simulink library "Actuator_Lib"  (Simulink 8.4)
settings: Solver=ode45  StartTime=0.0  StopTime=10.0  RelTol=1e-3
values from neighbouring files (symbols this model uses):
  AC = miniMUTT_rigid_config    [UAV_config.m]    (also in UAV_modelconfig.mat = )
  TrimCondition =     [UAV_trimcondition.mat]
undefined symbols (not defined in the file or in its folder): SampleTime
libraries: Actuator_Lib x31, simulink x7
settings Model: RequirementInfo="{}  %GIDa_26eb398f_e494_4241_9189_ccb3fdb74222"  Creator=austinmurch  LastModifiedBy=pseiler

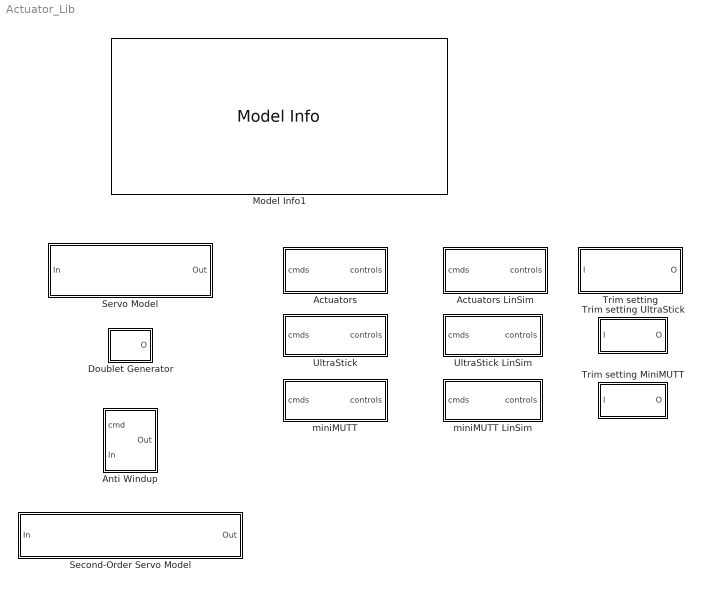
== system Actuator_Lib ==
  Actuators : Subsystem  BlockChoice=UltraStick  mask{aircraft=AC.aircraft}
      mask help: Set actuator models, either 'UltraStick120', 'UltraStick25e', or 'miniMUTT'
      mask init:
      | pathname = gcb;
      | 
      | switch lower(aircraft)
      |     case 'ultrastick120'
      |         set_param(pathname,'BlockChoice','UltraStick');
      |     case 'ultrastick25e'
      |         set_param(pathname,'BlockChoice','UltraStick');
      |     case 'minimutt'
      |         set_param(pathname,'BlockChoice','miniMUTT');
      |     case 'rigid_minimutt'
      |         set_param(pathname,'BlockChoice','miniMUTT');
      | end
      settings: TemplateBlock=self  MemberBlocks=UltraStick,miniMUTT
  Actuators LinSim : Subsystem  BlockChoice=miniMUTT LinSim  mask{aircraft=AC.aircraft}
      mask help: Set actuator models, either 'UltraStick120', 'UltraStick25e', or 'miniMUTT'
      mask init:
      | pathname = gcb;
      | 
      | switch lower(aircraft)
      |     case 'ultrastick120'
      |         set_param(pathname,'BlockChoice','UltraStick LinSim');
      |     case 'ultrastick25e'
      |         set_param(pathname,'BlockChoice','UltraStick LinSim');
      |     case 'minimutt'
      |         set_param(pathname,'BlockChoice','miniMUTT LinSim');
      |     case 'rigid_minimutt'
      |         set_param(pathname,'BlockChoice','miniMUTT LinSim');
      | end
      settings: TemplateBlock=self  MemberBlocks=UltraStick LinSim,miniMUTT LinSim
  Anti Windup : Subsystem  mask(Integrator Anti-Windup){MAX_DEF=0, MIN_DEF=0, gain_sign=off}
      mask prompts: MAX_DEF "Maximum surface deflection limit"; MIN_DEF "Minimum surface deflection limit"; gain_sign "Positive gains in control law"
      mask help:
      | This block uses boolean logic to eliminate integrator windup.
      | It compares the sign of the error between reference and output,
      | and the sign and position of the surface being controlled.
      mask Help:
      | See the "READ ME" block under the mask for a more thorough explanation of
      | how this block works.
  Doublet Generator : Subsystem  mask(DoubletGenerator){timeon=[3 10 17], pulsewidth=[2 2 2], amplitude=[0 0 0]}
      mask prompts: timeon "Time Start"; pulsewidth "Pulse Duration"
      mask help:
      | Doublet Generator.
      | Ouputs doublet of specificed amplitude and duration.
      |
      | If start/duration/amplitude parameters are vectors, then output is multichannel.
      mask Display: plot([.1 .3 .3001 .4 .4001 .5  .5001 .7],[0 0 1 1 -1 -1 0 0])
  Model Info1 : simulink/Model-Wide Utilities/Model Info  BlockCM=None  Frame=on  DisplayStringWithTags=|  HorizontalTextAlignment=Left  LeftAlignmentValue=0.02  SourceBlockDiagram=Actuator_Lib  TagMaxNumber=20
      | MODEL INFORMATION
      | Actuator Model Library
      | 
      | University of Minnesota
      | Aerospace Engineering and Mechanics
      | Copyright 2011 Regents of the University of Minnesota. All rights reserved.
      | 
      | == SVN Info ==
      | Last modified by %<LastModifiedBy> on %<LastModificationDate>
  Second-Order Servo Model : Subsystem  mask(Rate and Position Limited Servo){wn=10, zeta=1, RL=999, POS_hi=inf, POS_lo=-inf}
      mask prompts: wn "Natural Frequency, rad/sec"; zeta "Damping Ratio, unitless"; RL "Rate Limit:"; POS_hi "Position Limit High:"; POS_lo "Position Limit Low:"
      mask help: First order transfer function: w/(s+w), with rate and position limits.
      mask Help:
      | This block models a first order servo with the initial condition
      | on the integrator set to the steady state value for constant input.
      | The servo is rate and position limited and those values are set
      | in the block parameters.
      mask Display:
      | text(.48,.55,sprintf('wn=%3.1f rad/sec\n zeta= %3.1f',wn,zeta),'horizontalAlignment','center');
      | 
      | text(0.18,0.45,sprintf('|d/dt|\n<%0.1f',RL),'horizontalAlignment','center');
      | 
      | text(0.88,0.85,num2str(POS_hi),'horizontalAlignment', 'center');
      | text(0.88,0.2,num2str(POS_lo),'horizontalAlignment', 'center');
      | text(0.73,0.5,'P\nL');
      | 
      | 
      | plot([0.83 0.87 0.93 0.97],[0.4 0.4 0.6 0.6]);
      | plot([0.81 0.99],[0.5 0.5]);
      | plot([0.9 0.9],[0.3 0.7]);
      | plot([0.81 0.99 0.99 0.81 0.81],[0.3 0.3 0.7 0.7 0.3]);
  Servo Model : Subsystem  mask(Rate and Position Limited Servo){freq=10, RL=999.0, POS_hi=20.0, POS_lo=-30.0}
      mask prompts: freq "Bandwidth, Hz"; RL "Rate Limit:"; POS_hi "Position Limit High:"; POS_lo "Position Limit Low:"
      mask help: First order transfer function: w/(s+w), with rate and position limits.
      mask Help:
      | This block models a first order servo with the initial condition
      | on the integrator set to the steady state value for constant input.
      | The servo is rate and position limited and those values are set
      | in the block parameters.
      mask Display:
      | text(.48,.55,sprintf('%3.1f Hz\nBW',freq),'horizontalAlignment','center');
      | 
      | text(0.18,0.45,sprintf('|d/dt|\n<%0.1f',RL),'horizontalAlignment','center');
      | 
      | text(0.88,0.85,num2str(POS_hi),'horizontalAlignment', 'center');
      | text(0.88,0.2,num2str(POS_lo),'horizontalAlignment', 'center');
      | text(0.73,0.5,'P\nL');
      | 
      | 
      | plot([0.83 0.87 0.93 0.97],[0.4 0.4 0.6 0.6]);
      | plot([0.81 0.99],[0.5 0.5]);
      | plot([0.9 0.9],[0.3 0.7]);
      | plot([0.81 0.99 0.99 0.81 0.81],[0.3 0.3 0.7 0.7 0.3]);
  Trim setting : Subsystem  RequirementInfo="{}  %GIDa_fb3b993e_8e22_4fb1_9c4b_299134347a17"  BlockChoice=Trim setting UltraStick  mask{aircraft=AC.aircraft}
      mask prompts: aircraft "Aircraft model"
      mask init:
      | pathname = gcb;
      | 
      | switch lower(aircraft)
      |     case 'ultrastick120'
      |         set_param(pathname,'BlockChoice','Trim setting UltraStick');
      |     case 'ultrastick25e'
      |         set_param(pathname,'BlockChoice','Trim setting UltraStick');
      |     case 'minimutt'
      |         set_param(pathname,'BlockChoice','Trim setting MiniMUTT');
      |     case 'rigid_minimutt'
      |         set_param(pathname,'BlockChoice','Trim setting MiniMUTT');
      | end
      settings: TemplateBlock=self  MemberBlocks=Trim setting MiniMUTT,Trim setting UltraStick
  Trim setting MiniMUTT : Subsystem
  Trim setting UltraStick : Subsystem
  UltraStick : Subsystem
  UltraStick LinSim : Subsystem
  miniMUTT : Subsystem
  miniMUTT LinSim : Subsystem

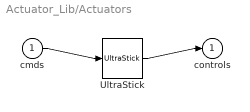
== system Actuator_Lib/Actuators ==
  cmds : Inport
  UltraStick : Actuator_Lib/UltraStick
  controls : Outport
  wires:
  cmds/1 -> UltraStick/1
  UltraStick/1 -> controls/1

== system Actuator_Lib/Actuators LinSim ==
  cmds : Inport
  miniMUTT LinSim : Actuator_Lib/miniMUTT LinSim
  controls : Outport
  wires:
  cmds/1 -> miniMUTT LinSim/1
  miniMUTT LinSim/1 -> controls/1

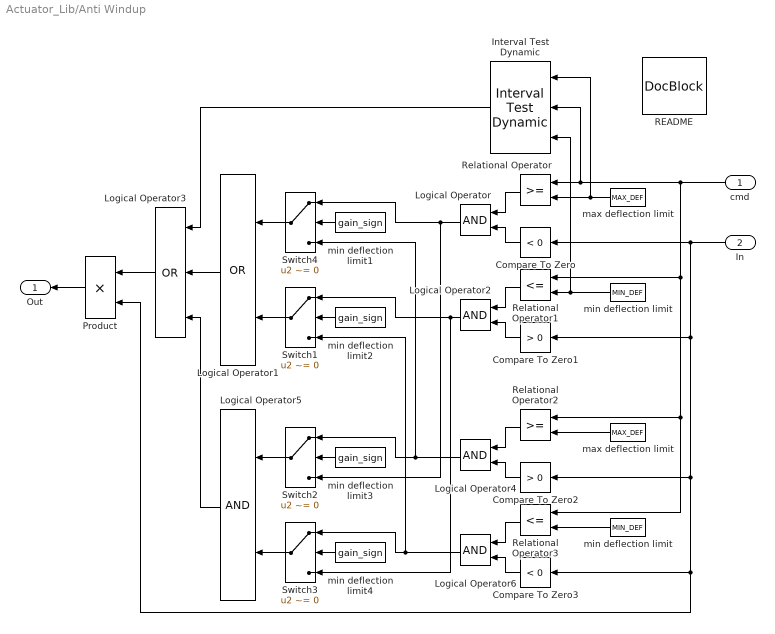
== system Actuator_Lib/Anti Windup ==
  cmd : Inport
  In : Inport  Port=2
  Compare To Zero : simulink/Logic and Bit Operations/Compare To Zero  relop=<  OutDataTypeStr=uint8
  Compare To Zero1 : simulink/Logic and Bit Operations/Compare To Zero  relop=>  OutDataTypeStr=uint8
  Compare To Zero2 : simulink/Logic and Bit Operations/Compare To Zero  relop=>  OutDataTypeStr=uint8
  Compare To Zero3 : simulink/Logic and Bit Operations/Compare To Zero  relop=<  OutDataTypeStr=uint8
  Interval Test Dynamic : simulink/Logic and Bit Operations/Interval Test Dynamic  IntervalClosedRight=on  IntervalClosedLeft=on  OutDataTypeStr=boolean
  Logical Operator{,2,4..6} (5 alike) : Logic  AllPortsSameDT=off  OutDataTypeStr=boolean  SampleTime=SampleTime
  Logical Operator1 : Logic  Operator=OR  AllPortsSameDT=off  OutDataTypeStr=boolean  SampleTime=SampleTime
  Logical Operator3 : Logic  Operator=OR  Inputs=3  AllPortsSameDT=off  OutDataTypeStr=boolean  SampleTime=SampleTime
  Product : Product  RndMeth=Zero
  README : simulink/Model-Wide Utilities/DocBlock  DocumentType=Text
  Relational Operator : RelationalOperator  OutDataTypeStr=boolean
  Relational Operator1 : RelationalOperator  Operator=<=  OutDataTypeStr=boolean
  Relational Operator2 : RelationalOperator  OutDataTypeStr=boolean
  Relational Operator3 : RelationalOperator  Operator=<=  OutDataTypeStr=boolean
  Switch{1..4} (4 alike) : Switch  Criteria=u2 ~= 0  SampleTime=SampleTime
  max deflection limit : Constant  Value=MAX_DEF  SampleTime=SampleTime
  "max deflection limit " : Constant  Value=MAX_DEF  SampleTime=SampleTime
  min deflection limit : Constant  Value=MIN_DEF  SampleTime=SampleTime
  "min deflection limit " : Constant  Value=MIN_DEF  SampleTime=SampleTime
  min deflection limit{1..4} (4 alike) : Constant  Value=gain_sign  SampleTime=SampleTime
  Out : Outport
  wires:
  Logical Operator5/1 -> Logical Operator3/3
  "max deflection limit "/1 -> Relational Operator2/2
  "min deflection limit "/1 -> Relational Operator3/2
  Relational Operator3/1 -> Logical Operator6/1
  Compare To Zero3/1 -> Logical Operator6/2
  Relational Operator2/1 -> Logical Operator4/1
  Compare To Zero2/1 -> Logical Operator4/2
  Interval Test Dynamic/1 -> Logical Operator3/1
  Logical Operator1/1 -> Logical Operator3/2
  Logical Operator3/1 -> Product/1
  Product/1 -> Out/1
  min deflection limit/1 -> Interval Test Dynamic/3, Relational Operator1/2
  Relational Operator1/1 -> Logical Operator2/1
  Compare To Zero1/1 -> Logical Operator2/2
  In/1 -> Product/2, Compare To Zero3/1, Compare To Zero2/1, Compare To Zero1/1, Compare To Zero/1
  Relational Operator/1 -> Logical Operator/1
  Compare To Zero/1 -> Logical Operator/2
  cmd/1 -> Relational Operator3/1, Relational Operator2/1, Relational Operator1/1, Interval Test Dynamic/2, Relational Operator/1
  max deflection limit/1 -> Interval Test Dynamic/1, Relational Operator/2
  min deflection limit2/1 -> Switch1/2
  min deflection limit3/1 -> Switch2/2
  min deflection limit4/1 -> Switch3/2
  Switch2/1 -> Logical Operator5/1
  Switch3/1 -> Logical Operator5/2
  Switch1/1 -> Logical Operator1/2
  Switch4/1 -> Logical Operator1/1
  min deflection limit1/1 -> Switch4/2
  Logical Operator/1 -> Switch4/1, Switch2/3
  Logical Operator2/1 -> Switch1/1, Switch3/3
  Logical Operator4/1 -> Switch2/1, Switch4/3
  Logical Operator6/1 -> Switch3/1, Switch1/3

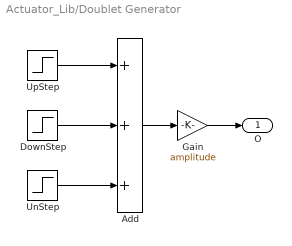
== system Actuator_Lib/Doublet Generator ==
  Add : Sum  Inputs=+++
  DownStep : Step  Time=timeon+pulsewidth  After=-2  SampleTime=0
  Gain : Gain  Gain=amplitude
  UnStep : Step  Time=timeon+2*pulsewidth  SampleTime=0
  UpStep : Step  Time=timeon  SampleTime=0
  O : Outport
  wires:
  Gain/1 -> O/1
  Add/1 -> Gain/1
  UnStep/1 -> Add/3
  DownStep/1 -> Add/2
  UpStep/1 -> Add/1

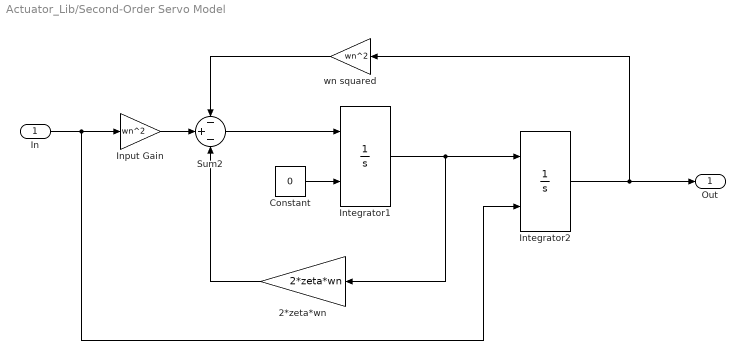
== system Actuator_Lib/Second-Order Servo Model ==
  In : Inport
  2*zeta*wn : Gain  Gain=2*zeta*wn
  Constant : Constant  Value=0
  Input Gain : Gain  Gain=wn^2
  Integrator1 : Integrator  InitialConditionSource=external  LimitOutput=on  UpperSaturationLimit=RL  LowerSaturationLimit=-RL  IgnoreLimit=on
  Integrator2 : Integrator  InitialConditionSource=external  LimitOutput=on  UpperSaturationLimit=POS_hi  LowerSaturationLimit=POS_lo  IgnoreLimit=on
  Sum2 : Sum  Inputs=-+-
  wn squared : Gain  Gain=wn^2
  Out : Outport  PortDimensions=1
  wires:
  In/1 -> Input Gain/1, Integrator2/2
  Input Gain/1 -> Sum2/2
  2*zeta*wn/1 -> Sum2/3
  Constant/1 -> Integrator1/2
  Sum2/1 -> Integrator1/1
  Integrator1/1 -> Integrator2/1, 2*zeta*wn/1
  wn squared/1 -> Sum2/1
  Integrator2/1 -> Out/1, wn squared/1

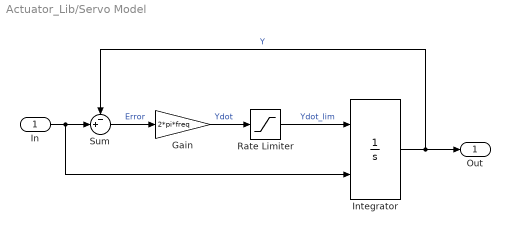
== system Actuator_Lib/Servo Model ==
  In : Inport
  Gain : Gain  Gain=2*pi*freq  SaturateOnIntegerOverflow=on  OutDataTypeStr=Inherit: Same as input  ParamDataTypeStr=Inherit: Same as input
  Integrator : Integrator  InitialConditionSource=external  LimitOutput=on  UpperSaturationLimit=POS_hi  LowerSaturationLimit=POS_lo  IgnoreLimit=on
  Rate Limiter : Saturate  UpperLimit=RL  LowerLimit=-RL
  Sum : Sum  Inputs=-+|  SaturateOnIntegerOverflow=on  InputSameDT=on  OutDataTypeStr=Inherit: Same as first input
  Out : Outport  PortDimensions=1
  wires:
  Gain/1 -> Rate Limiter/1  "Ydot"
  Sum/1 -> Gain/1  "Error"
  Integrator/1 -> Sum/1, Out/1  "Y"
  Rate Limiter/1 -> Integrator/1  "Ydot_lim"
  In/1 -> Integrator/2, Sum/2

== system Actuator_Lib/Trim setting ==
  I : Inport
  Trim setting UltraStick : Actuator_Lib/Trim setting UltraStick
  O : Outport
  wires:
  I/1 -> Trim setting UltraStick/1
  Trim setting UltraStick/1 -> O/1

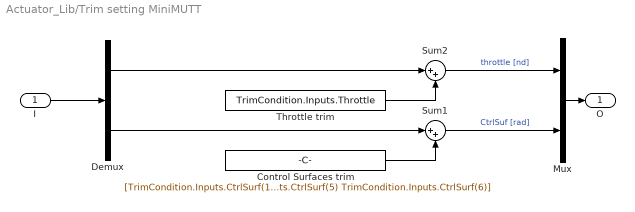
== system Actuator_Lib/Trim setting MiniMUTT ==
  I : Inport
  Control Surfaces trim : Constant  Value=[TrimCondition.Inputs.CtrlSurf(1) TrimCondition.Inputs.CtrlSurf(2) TrimCondition.Inputs.CtrlSurf(3) TrimCondition.Inputs.CtrlSurf(4) TrimCondition.Inputs.CtrlSurf(5) TrimCondition.Inputs.CtrlSurf(6)]
  Demux : Demux  Outputs=[1 ,-1]
  Mux : Mux  Inputs=2
  Sum1 : Sum  Inputs=|++
  Sum2 : Sum  Inputs=|++
  Throttle trim : Constant  Value=TrimCondition.Inputs.Throttle
  O : Outport
  wires:
  Sum1/1 -> Mux/2  "CtrlSuf [rad]"
  Demux/1 -> Sum2/1
  Sum2/1 -> Mux/1  "throttle [nd]"
  Throttle trim/1 -> Sum2/2
  Control Surfaces trim/1 -> Sum1/2
  I/1 -> Demux/1
  Demux/2 -> Sum1/1
  Mux/1 -> O/1

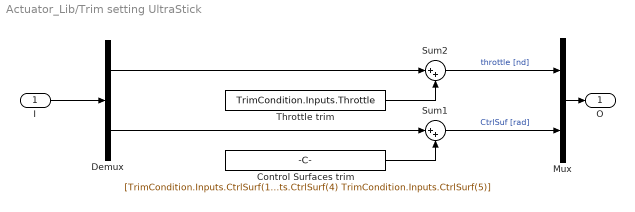
== system Actuator_Lib/Trim setting UltraStick ==
  I : Inport
  Control Surfaces trim : Constant  Value=[TrimCondition.Inputs.CtrlSurf(1) TrimCondition.Inputs.CtrlSurf(2) TrimCondition.Inputs.CtrlSurf(3)*-1 TrimCondition.Inputs.CtrlSurf(3) TrimCondition.Inputs.CtrlSurf(4) TrimCondition.Inputs.CtrlSurf(5)]
  Demux : Demux  Outputs=[1 ,-1]
  Mux : Mux  Inputs=2
  Sum1 : Sum  Inputs=|++
  Sum2 : Sum  Inputs=|++
  Throttle trim : Constant  Value=TrimCondition.Inputs.Throttle
  O : Outport
  wires:
  Sum1/1 -> Mux/2  "CtrlSuf [rad]"
  Demux/1 -> Sum2/1
  Sum2/1 -> Mux/1  "throttle [nd]"
  Throttle trim/1 -> Sum2/2
  Control Surfaces trim/1 -> Sum1/2
  I/1 -> Demux/1
  Demux/2 -> Sum1/1
  Mux/1 -> O/1

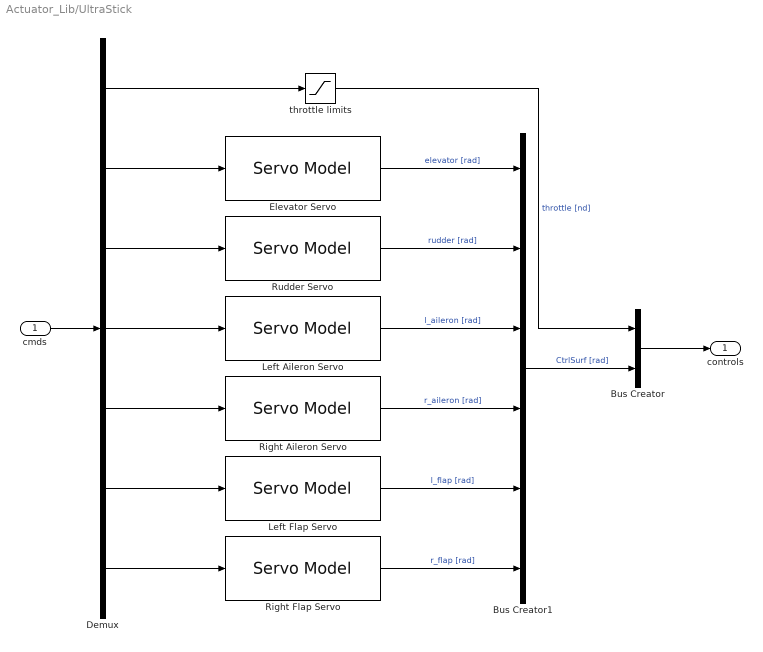
== system Actuator_Lib/UltraStick ==
  cmds : Inport
  Bus Creator : BusCreator  Inputs=2
  Bus Creator1 : BusCreator  Inputs=6
  Demux : Demux  Outputs=7
  Elevator Servo : Actuator_Lib/Servo Model  freq=AC.Actuator.elevator.BW  RL=AC.Actuator.elevator.RateLim  POS_hi=AC.Actuator.elevator.PosLim  POS_lo=AC.Actuator.elevator.NegLim
  Left Aileron Servo : Actuator_Lib/Servo Model  freq=AC.Actuator.l_aileron.BW  RL=AC.Actuator.l_aileron.RateLim  POS_hi=AC.Actuator.l_aileron.PosLim  POS_lo=AC.Actuator.l_aileron.NegLim
  Left Flap Servo : Actuator_Lib/Servo Model  freq=AC.Actuator.l_flap.BW  RL=AC.Actuator.l_flap.RateLim  POS_hi=AC.Actuator.l_flap.PosLim  POS_lo=AC.Actuator.l_flap.NegLim
  Right Aileron Servo : Actuator_Lib/Servo Model  freq=AC.Actuator.r_aileron.BW  RL=AC.Actuator.r_aileron.RateLim  POS_hi=AC.Actuator.r_aileron.PosLim  POS_lo=AC.Actuator.r_aileron.NegLim
  Right Flap Servo : Actuator_Lib/Servo Model  freq=AC.Actuator.l_flap.BW  RL=AC.Actuator.l_flap.RateLim  POS_hi=AC.Actuator.l_flap.PosLim  POS_lo=AC.Actuator.l_flap.NegLim
  Rudder Servo : Actuator_Lib/Servo Model  freq=AC.Actuator.rudder.BW  RL=AC.Actuator.rudder.RateLim  POS_hi=AC.Actuator.rudder.PosLim  POS_lo=AC.Actuator.rudder.NegLim
  throttle limits : Saturate  UpperLimit=AC.Actuator.throttle.PosLim  LowerLimit=AC.Actuator.throttle.NegLim
  controls : Outport
  wires:
  Demux/5 -> Right Aileron Servo/1
  Demux/7 -> Right Flap Servo/1
  Right Flap Servo/1 -> Bus Creator1/6  "r_flap [rad]"
  Right Aileron Servo/1 -> Bus Creator1/4  "r_aileron [rad]"
  Left Flap Servo/1 -> Bus Creator1/5  "l_flap [rad]"
  Demux/6 -> Left Flap Servo/1
  Left Aileron Servo/1 -> Bus Creator1/3  "l_aileron [rad]"
  Demux/4 -> Left Aileron Servo/1
  Rudder Servo/1 -> Bus Creator1/2  "rudder [rad]"
  Demux/3 -> Rudder Servo/1
  Elevator Servo/1 -> Bus Creator1/1  "elevator [rad]"
  Demux/2 -> Elevator Servo/1
  throttle limits/1 -> Bus Creator/1  "throttle [nd]"
  Demux/1 -> throttle limits/1
  cmds/1 -> Demux/1
  Bus Creator/1 -> controls/1
  Bus Creator1/1 -> Bus Creator/2  "CtrlSurf [rad]"

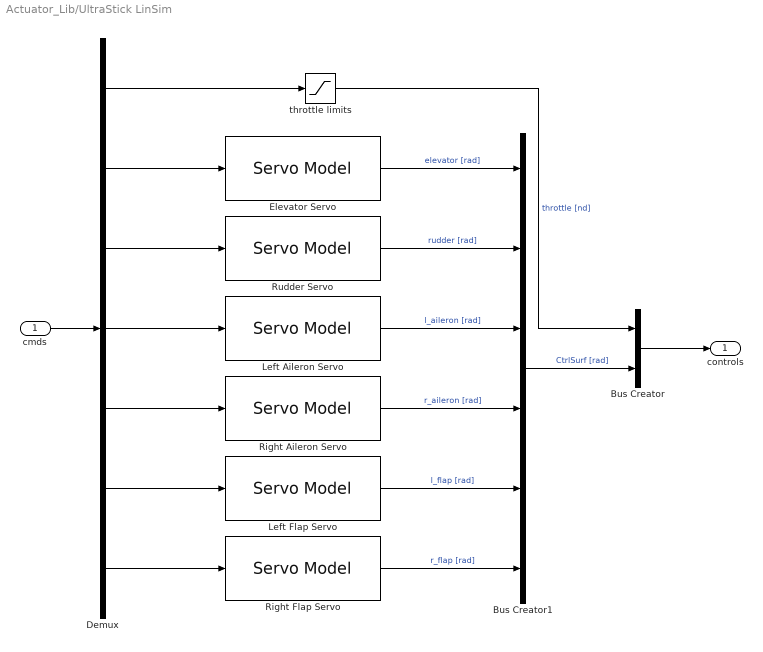
== system Actuator_Lib/UltraStick LinSim ==
  cmds : Inport
  Bus Creator : BusCreator  Inputs=2
  Bus Creator1 : BusCreator  Inputs=6
  Demux : Demux  Outputs=7
  Elevator Servo : Actuator_Lib/Servo Model  freq=AC.Actuator.elevator.BW  RL=AC.Actuator.elevator.RateLim  POS_hi=AC.Actuator.elevator.PosLim-TrimCondition.Inputs.CtrlSurf(1)  POS_lo=AC.Actuator.elevator.NegLim-TrimCondition.Inputs.CtrlSurf(1)
  Left Aileron Servo : Actuator_Lib/Servo Model  freq=AC.Actuator.l_aileron.BW  RL=AC.Actuator.l_aileron.RateLim  POS_hi=AC.Actuator.l_aileron.PosLim+TrimCondition.Inputs.CtrlSurf(3)  POS_lo=AC.Actuator.l_aileron.NegLim+-TrimCondition.Inputs.CtrlSurf(3)
  Left Flap Servo : Actuator_Lib/Servo Model  freq=AC.Actuator.l_flap.BW  RL=AC.Actuator.l_flap.RateLim  POS_hi=AC.Actuator.l_flap.PosLim-TrimCondition.Inputs.CtrlSurf(4)  POS_lo=AC.Actuator.l_flap.NegLim-TrimCondition.Inputs.CtrlSurf(4)
  Right Aileron Servo : Actuator_Lib/Servo Model  freq=AC.Actuator.r_aileron.BW  RL=AC.Actuator.r_aileron.RateLim  POS_hi=AC.Actuator.r_aileron.PosLim--TrimCondition.Inputs.CtrlSurf(3)  POS_lo=AC.Actuator.r_aileron.NegLim--TrimCondition.Inputs.CtrlSurf(3)
  Right Flap Servo : Actuator_Lib/Servo Model  freq=AC.Actuator.l_flap.BW  RL=AC.Actuator.l_flap.RateLim  POS_hi=AC.Actuator.l_flap.PosLim-TrimCondition.Inputs.CtrlSurf(5)  POS_lo=AC.Actuator.l_flap.NegLim-TrimCondition.Inputs.CtrlSurf(5)
  Rudder Servo : Actuator_Lib/Servo Model  freq=AC.Actuator.rudder.BW  RL=AC.Actuator.rudder.RateLim  POS_hi=AC.Actuator.rudder.PosLim-TrimCondition.Inputs.CtrlSurf(2)  POS_lo=AC.Actuator.rudder.NegLim-TrimCondition.Inputs.CtrlSurf(2)
  throttle limits : Saturate  UpperLimit=AC.Actuator.throttle.PosLim-TrimCondition.Inputs.Throttle  LowerLimit=AC.Actuator.throttle.NegLim-TrimCondition.Inputs.Throttle
  controls : Outport
  wires:
  Demux/5 -> Right Aileron Servo/1
  Demux/7 -> Right Flap Servo/1
  Right Flap Servo/1 -> Bus Creator1/6  "r_flap [rad]"
  Right Aileron Servo/1 -> Bus Creator1/4  "r_aileron [rad]"
  Left Flap Servo/1 -> Bus Creator1/5  "l_flap [rad]"
  Demux/6 -> Left Flap Servo/1
  Left Aileron Servo/1 -> Bus Creator1/3  "l_aileron [rad]"
  Demux/4 -> Left Aileron Servo/1
  Rudder Servo/1 -> Bus Creator1/2  "rudder [rad]"
  Demux/3 -> Rudder Servo/1
  Elevator Servo/1 -> Bus Creator1/1  "elevator [rad]"
  Demux/2 -> Elevator Servo/1
  throttle limits/1 -> Bus Creator/1  "throttle [nd]"
  Demux/1 -> throttle limits/1
  cmds/1 -> Demux/1
  Bus Creator/1 -> controls/1
  Bus Creator1/1 -> Bus Creator/2  "CtrlSurf [rad]"

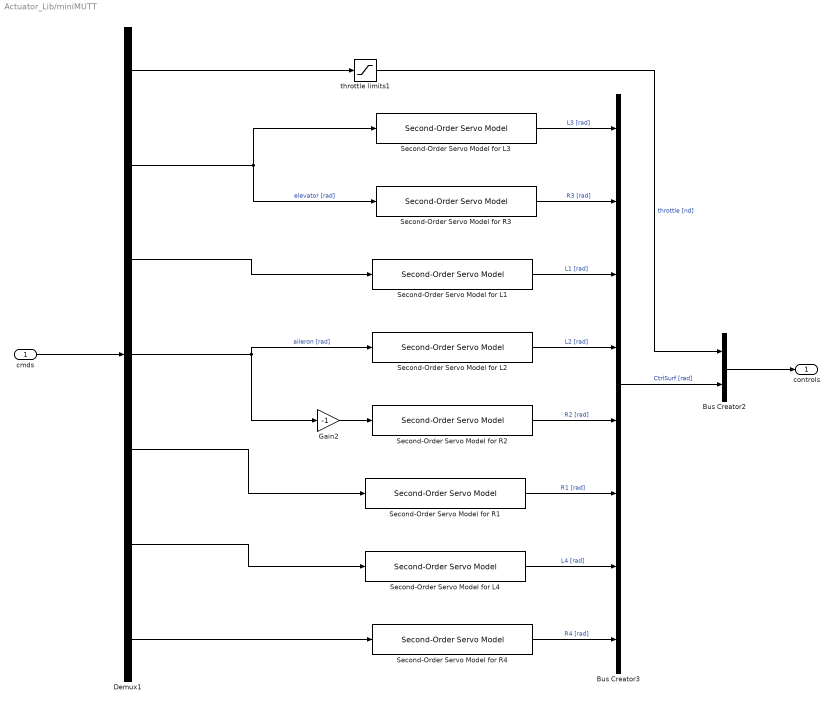
== system Actuator_Lib/miniMUTT ==
  cmds : Inport
  Bus Creator2 : BusCreator  Inputs=2
  Bus Creator3 : BusCreator  Inputs=8
  Demux1 : Demux  Outputs=7
  Gain2 : Gain  Gain=-1
  Second-Order Servo Model for L1 : Actuator_Lib/Second-Order Servo Model  wn=AC.Actuator.L1.wn  zeta=AC.Actuator.L1.zeta  RL=AC.Actuator.L1.RateLim  POS_hi=AC.Actuator.L1.PosLim  POS_lo=AC.Actuator.L1.NegLim
  Second-Order Servo Model for L2 : Actuator_Lib/Second-Order Servo Model  wn=AC.Actuator.L2.wn  zeta=AC.Actuator.L2.zeta  RL=AC.Actuator.L2.RateLim  POS_hi=AC.Actuator.L2.PosLim  POS_lo=AC.Actuator.L2.NegLim
  Second-Order Servo Model for L3 : Actuator_Lib/Second-Order Servo Model  wn=AC.Actuator.L3.wn  zeta=AC.Actuator.L3.zeta  RL=AC.Actuator.L3.RateLim  POS_hi=AC.Actuator.L3.PosLim  POS_lo=AC.Actuator.L3.NegLim
  Second-Order Servo Model for L4 : Actuator_Lib/Second-Order Servo Model  wn=AC.Actuator.L4.wn  zeta=AC.Actuator.L4.zeta  RL=AC.Actuator.L4.RateLim  POS_hi=AC.Actuator.L4.PosLim  POS_lo=AC.Actuator.L4.NegLim
  Second-Order Servo Model for R1 : Actuator_Lib/Second-Order Servo Model  wn=AC.Actuator.R1.wn  zeta=AC.Actuator.R1.zeta  RL=AC.Actuator.R1.RateLim  POS_hi=AC.Actuator.R1.PosLim  POS_lo=AC.Actuator.R1.NegLim
  Second-Order Servo Model for R2 : Actuator_Lib/Second-Order Servo Model  wn=AC.Actuator.R2.wn  zeta=AC.Actuator.R2.zeta  RL=AC.Actuator.R2.RateLim  POS_hi=AC.Actuator.R2.PosLim  POS_lo=AC.Actuator.R2.NegLim
  Second-Order Servo Model for R3 : Actuator_Lib/Second-Order Servo Model  wn=AC.Actuator.R3.wn  zeta=AC.Actuator.R3.zeta  RL=AC.Actuator.R3.RateLim  POS_hi=AC.Actuator.R3.PosLim  POS_lo=AC.Actuator.R3.NegLim
  Second-Order Servo Model for R4 : Actuator_Lib/Second-Order Servo Model  wn=AC.Actuator.R4.wn  zeta=AC.Actuator.R4.zeta  RL=AC.Actuator.R4.RateLim  POS_hi=AC.Actuator.R4.PosLim  POS_lo=AC.Actuator.R4.NegLim
  throttle limits1 : Saturate  UpperLimit=AC.Actuator.throttle.PosLim  LowerLimit=AC.Actuator.throttle.NegLim
  controls : Outport
  wires:
  throttle limits1/1 -> Bus Creator2/1  "throttle [nd]"
  Demux1/1 -> throttle limits1/1
  Bus Creator2/1 -> controls/1
  Bus Creator3/1 -> Bus Creator2/2  "CtrlSurf [rad]"
  cmds/1 -> Demux1/1
  Second-Order Servo Model for L3/1 -> Bus Creator3/1  "L3 [rad]"
  Second-Order Servo Model for R3/1 -> Bus Creator3/2  "R3 [rad]"
  Demux1/2 -> Second-Order Servo Model for R3/1, Second-Order Servo Model for L3/1  "elevator [rad]"
  Second-Order Servo Model for L1/1 -> Bus Creator3/3  "L1 [rad]"
  Demux1/3 -> Second-Order Servo Model for L1/1
  Second-Order Servo Model for L2/1 -> Bus Creator3/4  "L2 [rad]"
  Second-Order Servo Model for R2/1 -> Bus Creator3/5  "R2 [rad]"
  Gain2/1 -> Second-Order Servo Model for R2/1
  Demux1/4 -> Second-Order Servo Model for L2/1, Gain2/1  "aileron [rad]"
  Second-Order Servo Model for R4/1 -> Bus Creator3/8  "R4 [rad]"
  Demux1/7 -> Second-Order Servo Model for R4/1
  Second-Order Servo Model for L4/1 -> Bus Creator3/7  "L4 [rad]"
  Demux1/6 -> Second-Order Servo Model for L4/1
  Second-Order Servo Model for R1/1 -> Bus Creator3/6  "R1 [rad]"
  Demux1/5 -> Second-Order Servo Model for R1/1

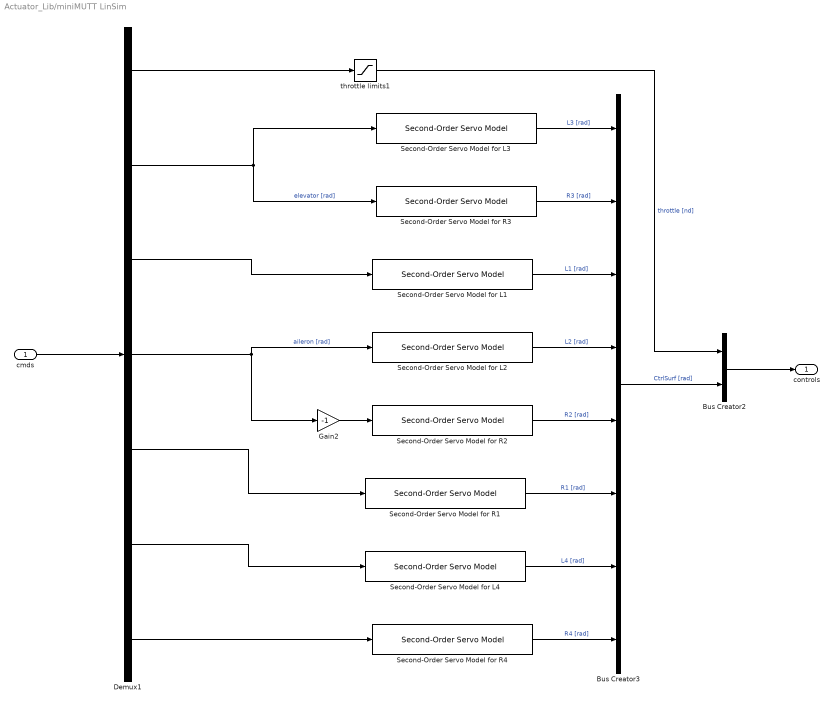
== system Actuator_Lib/miniMUTT LinSim ==
  cmds : Inport
  Bus Creator2 : BusCreator  Inputs=2
  Bus Creator3 : BusCreator  Inputs=8
  Demux1 : Demux  Outputs=7
  Gain2 : Gain  Gain=-1
  Second-Order Servo Model for L1 : Actuator_Lib/Second-Order Servo Model  wn=AC.Actuator.L1.wn  zeta=AC.Actuator.L1.zeta  RL=AC.Actuator.L1.RateLim  POS_hi=AC.Actuator.L1.PosLim-TrimCondition.Inputs.CtrlSurf(2)  POS_lo=AC.Actuator.L1.NegLim-TrimCondition.Inputs.CtrlSurf(2)
  Second-Order Servo Model for L2 : Actuator_Lib/Second-Order Servo Model  wn=AC.Actuator.L2.wn  zeta=AC.Actuator.L2.zeta  RL=AC.Actuator.L2.RateLim  POS_hi=AC.Actuator.L2.PosLim-TrimCondition.Inputs.CtrlSurf(3)  POS_lo=AC.Actuator.L2.NegLim-TrimCondition.Inputs.CtrlSurf(3)
  Second-Order Servo Model for L3 : Actuator_Lib/Second-Order Servo Model  wn=AC.Actuator.L3.wn  zeta=AC.Actuator.L3.zeta  RL=AC.Actuator.L3.RateLim  POS_hi=AC.Actuator.L3.PosLim-TrimCondition.Inputs.CtrlSurf(1)  POS_lo=AC.Actuator.L3.NegLim-TrimCondition.Inputs.CtrlSurf(1)
  Second-Order Servo Model for L4 : Actuator_Lib/Second-Order Servo Model  wn=AC.Actuator.L4.wn  zeta=AC.Actuator.L4.zeta  RL=AC.Actuator.L4.RateLim  POS_hi=AC.Actuator.L4.PosLim-TrimCondition.Inputs.CtrlSurf(5)  POS_lo=AC.Actuator.L4.NegLim-TrimCondition.Inputs.CtrlSurf(5)
  Second-Order Servo Model for R1 : Actuator_Lib/Second-Order Servo Model  wn=AC.Actuator.R1.wn  zeta=AC.Actuator.R1.zeta  RL=AC.Actuator.R1.RateLim  POS_hi=AC.Actuator.R1.PosLim-TrimCondition.Inputs.CtrlSurf(4)  POS_lo=AC.Actuator.R1.NegLim-TrimCondition.Inputs.CtrlSurf(4)
  Second-Order Servo Model for R2 : Actuator_Lib/Second-Order Servo Model  wn=AC.Actuator.R2.wn  zeta=AC.Actuator.R2.zeta  RL=AC.Actuator.R2.RateLim  POS_hi=AC.Actuator.R2.PosLim+TrimCondition.Inputs.CtrlSurf(3)  POS_lo=AC.Actuator.R2.NegLim+TrimCondition.Inputs.CtrlSurf(3)
  Second-Order Servo Model for R3 : Actuator_Lib/Second-Order Servo Model  wn=AC.Actuator.R3.wn  zeta=AC.Actuator.R3.zeta  RL=AC.Actuator.R3.RateLim  POS_hi=AC.Actuator.R3.PosLim-TrimCondition.Inputs.CtrlSurf(1)  POS_lo=AC.Actuator.R3.NegLim-TrimCondition.Inputs.CtrlSurf(1)
  Second-Order Servo Model for R4 : Actuator_Lib/Second-Order Servo Model  wn=AC.Actuator.R4.wn  zeta=AC.Actuator.R4.zeta  RL=AC.Actuator.R4.RateLim  POS_hi=AC.Actuator.R4.PosLim-TrimCondition.Inputs.CtrlSurf(6)  POS_lo=AC.Actuator.R4.NegLim-TrimCondition.Inputs.CtrlSurf(6)
  throttle limits1 : Saturate  UpperLimit=AC.Actuator.throttle.PosLim-TrimCondition.Inputs.Throttle  LowerLimit=AC.Actuator.throttle.NegLim-TrimCondition.Inputs.Throttle
  controls : Outport
  wires:
  throttle limits1/1 -> Bus Creator2/1  "throttle [nd]"
  Demux1/1 -> throttle limits1/1
  Bus Creator2/1 -> controls/1
  Bus Creator3/1 -> Bus Creator2/2  "CtrlSurf [rad]"
  cmds/1 -> Demux1/1
  Second-Order Servo Model for L3/1 -> Bus Creator3/1  "L3 [rad]"
  Second-Order Servo Model for R3/1 -> Bus Creator3/2  "R3 [rad]"
  Demux1/2 -> Second-Order Servo Model for R3/1, Second-Order Servo Model for L3/1  "elevator [rad]"
  Second-Order Servo Model for L1/1 -> Bus Creator3/3  "L1 [rad]"
  Demux1/3 -> Second-Order Servo Model for L1/1
  Second-Order Servo Model for L2/1 -> Bus Creator3/4  "L2 [rad]"
  Second-Order Servo Model for R2/1 -> Bus Creator3/5  "R2 [rad]"
  Gain2/1 -> Second-Order Servo Model for R2/1
  Demux1/4 -> Second-Order Servo Model for L2/1, Gain2/1  "aileron [rad]"
  Second-Order Servo Model for R4/1 -> Bus Creator3/8  "R4 [rad]"
  Demux1/7 -> Second-Order Servo Model for R4/1
  Second-Order Servo Model for L4/1 -> Bus Creator3/7  "L4 [rad]"
  Demux1/6 -> Second-Order Servo Model for L4/1
  Second-Order Servo Model for R1/1 -> Bus Creator3/6  "R1 [rad]"
  Demux1/5 -> Second-Order Servo Model for R1/1
